simulink model "ForceField"  (R2022b)
settings: Solver=FixedStepDiscrete  StartTime=0.0  StopTime=inf  FixedStep=0.001  RelTol=1e-3
libraries: PhanTorque_3Dof_Library_64Bits x2, simulink x1
settings Model: Creator=carlos.aldana  LastModifiedBy=bioen
settings SolverCC: AlgebraicLoopSolver=TrustRegion
settings DataIOCC: LimitDataPoints=on  SaveFormat=Array  ReturnWorkspaceOutputs=off
settings OptimizationCC: BlockReduction=off  BooleanDataType=off  LifeSpan=inf
settings DebuggingCC: SaveWithParameterizedLinksMsg=none  UnderspecifiedInitializationDetection=Classic  MergeDetectMultiDrivingBlocksExec=none  SignalResolutionControl=TryResolveAllWithWarning  UnconnectedInputMsg=warning  UnconnectedOutputMsg=warning  UnconnectedLineMsg=warning  AllowSymbolicDim=off  SFUnexpectedBacktrackingDiag=warning  SFNoUnconditionalDefaultTransitionDiag=warning  SFExecutionAtInitializationDiag=none  SFMachineParentedDataDiag=warning  ArithmeticOperatorsInVariantConditions=warning
settings HardwareCC: ProdBitPerPointer=32  ProdBitPerSizeT=32  ProdBitPerPtrDiffT=32  ProdLargestAtomicFloat=None  ProdIntDivRoundTo=Undefined  ProdEndianess=Unspecified  ProdWordSize=32  ProdHWDeviceType=32-bit Generic  TargetUnknown=on
settings ModelReferenceCC: EnableRefExpFcnMdlSchedulingChecks=on  PropagateSignalLabelsOutOfModel=off
settings SFSimCC: SimUseLocalCustomCode=off  CustomCodeUndefinedFunction=UseInterfaceOnly
settings RTWCC: RTWUseLocalCustomCode=off  DLArmComputeVersion=19.05
settings CodeAppCC: StateflowObjectComments=on
settings GRTTargetCC: TargetLangStandard=C89/C90 (ANSI)
settings ConfigComp: CovMetricSettings=dw  CovSaveCumulativeToWorkspaceVar=on  CovSaveSingleToWorkspaceVar=on  CovExternalEMLEnable=off  CovSFcnEnable=off

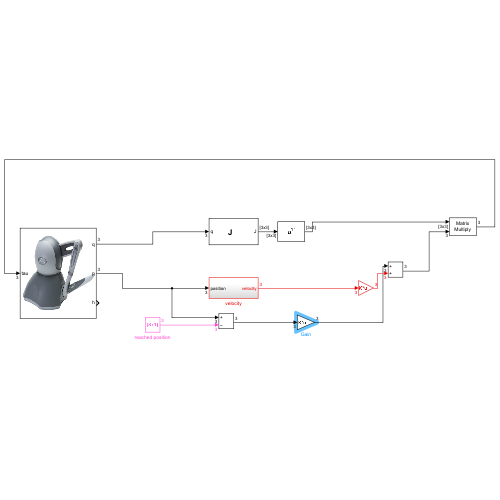
[thumbnail: Simulink's stored preview of the top-level diagram]
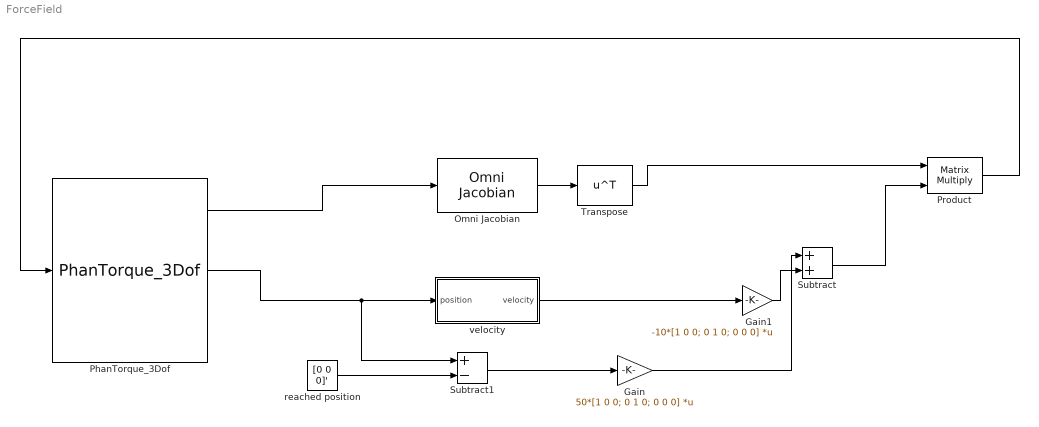
== system ForceField ==
  Gain : Gain  Gain=50*[1 0 0; 0 1 0; 0 0 0]  Multiplication=Matrix(K*u)
  Gain1 : Gain  Gain=-10*[1 0 0; 0 1 0; 0 0 0]  Multiplication=Matrix(K*u)
  Omni Jacobian : PhanTorque_3Dof_Library_64Bits/Omni Jacobian  SystemSampleTime=-1  VariantActivationTime=update diagram  Latency=0  AutoFrameSizeCalculation=off
  PhanTorque_3Dof : PhanTorque_3Dof_Library_64Bits/PhanTorque_3Dof  Haptic_Name='Default Device'
  Product : Product  Multiplication=Matrix(*)
  Subtract : Sum
  Subtract1 : Sum  Inputs=+-
  Transpose : Math  Operator=transpose  SignedPower=on
  reached position : Constant  Value=[0 0 0]'
  velocity : Subsystem
  wires:
  PhanTorque_3Dof/1 -> Omni Jacobian/1
  Omni Jacobian/1 -> Transpose/1
  PhanTorque_3Dof/2 -> Subtract1/1, velocity/1(position)
  Transpose/1 -> Product/1
  Gain/1 -> Subtract/1
  Gain1/1 -> Subtract/2
  Subtract/1 -> Product/2
  velocity/1(velocity) -> Gain1/1
  Product/1 -> PhanTorque_3Dof/1
  reached position/1 -> Subtract1/2
  Subtract1/1 -> Gain/1

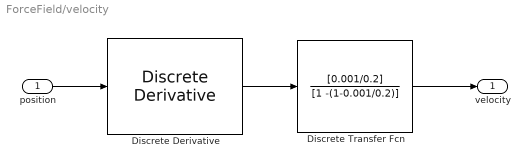
== system ForceField/velocity ==
  position : Inport
  Discrete Derivative : simulink/Discrete/Discrete Derivative  gainval=1.0  ICPrevScaledInput=0.0  OutMin=[]  OutMax=[]  OutDataType=fixdt(1, 16)  OutScaling=2^-10  DoSatur=off
  Discrete Transfer Fcn : DiscreteTransferFcn  Numerator=[0.001/0.2]  Denominator=[1 -(1-0.001/0.2)]
  velocity : Outport  VectorParamsAs1DForOutWhenUnconnected=off
  wires:
  position/1 -> Discrete Derivative/1
  Discrete Derivative/1 -> Discrete Transfer Fcn/1
  Discrete Transfer Fcn/1 -> velocity/1
